simulink model "Test_Decoder_3_to_8"  (R2023a)
settings: Solver=ode45  StartTime=0.0  StopTime=len  RelTol=1e-3  EnableMultiTasking=on
libraries: simulink x2, Decoders_Lib x1
settings Model: Creator=N  LastModifiedBy=Jozko Mrkvicka
settings SolverCC: AlgebraicLoopSolver=TrustRegion
settings DataIOCC: SaveFormat=Array  ReturnWorkspaceOutputs=off
settings OptimizationCC: LifeSpan=inf
settings DebuggingCC: UnconnectedInputMsg=warning  UnconnectedOutputMsg=warning  UnconnectedLineMsg=warning  SFUnexpectedBacktrackingDiag=warning  SFNoUnconditionalDefaultTransitionDiag=warning  SFExecutionAtInitializationDiag=none  ArithmeticOperatorsInVariantConditions=warning
settings HardwareCC: ProdWordSize=32
settings SFSimCC: SimUseLocalCustomCode=off  CustomCodeUndefinedFunction=UseInterfaceOnly
settings RTWCC: RTWUseLocalCustomCode=off
settings CodeAppCC: StateflowObjectComments=on
settings GRTTargetCC: TargetLangStandard=C89/C90 (ANSI)
settings ConfigComp: CovMetricSettings=dw  CovSaveCumulativeToWorkspaceVar=on  CovSaveSingleToWorkspaceVar=on  CovExternalEMLEnable=off

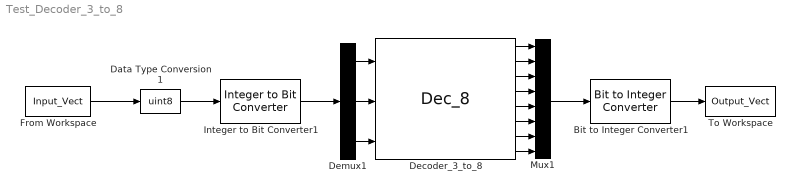
== system Test_Decoder_3_to_8 ==
  Bit to Integer Converter1 : simulink/Logic and Bit Operations/Bit to Integer Converter  nbits=8  bitOrder=MSB first  signedOutputValues=Unsigned  outDtype=uint8  outDtypeSigned=Inherit via internal rule
      settings: LibrarySourceBlock=|
      | commutil2/Bit to Integer
      | Converter
  Data Type Conversion1 : DataTypeConversion  OutDataTypeStr=uint8  SaturateOnIntegerOverflow=off  RndMeth=Floor
  Decoder_3_to_8 : Decoders_Lib/Dec_8  SystemSampleTime=-1  VariantActivationTime=update diagram  Latency=0  AutoFrameSizeCalculation=off
  Demux1 : Demux  Outputs=3
  From Workspace : FromWorkspace  VariableName=Input_Vect  SampleTime=1  Interpolate=off  ZeroCross=off  OutputAfterFinalValue=Holding final value
  Integer to Bit Converter1 : simulink/Logic and Bit Operations/Integer to Bit Converter  nbits=3  signedInputValues=Unsigned  bitOrder=MSB first  outDtype=uint8
      settings: LibrarySourceBlock=|
      | commutil2/Integer to Bit
      | Converter
  Mux1 : Mux  Inputs=8
  To Workspace : ToWorkspace  VariableName=Output_Vect  SampleTime=1
  wires:
  Decoder_3_to_8/1 -> Mux1/1
  Decoder_3_to_8/8 -> Mux1/8
  Decoder_3_to_8/7 -> Mux1/7
  Decoder_3_to_8/6 -> Mux1/6
  Decoder_3_to_8/5 -> Mux1/5
  Decoder_3_to_8/4 -> Mux1/4
  Decoder_3_to_8/3 -> Mux1/3
  Decoder_3_to_8/2 -> Mux1/2
  Mux1/1 -> Bit to Integer Converter1/1
  Demux1/2 -> Decoder_3_to_8/2
  Demux1/3 -> Decoder_3_to_8/3
  Demux1/1 -> Decoder_3_to_8/1
  Integer to Bit Converter1/1 -> Demux1/1
  Data Type Conversion1/1 -> Integer to Bit Converter1/1
  From Workspace/1 -> Data Type Conversion1/1
  Bit to Integer Converter1/1 -> To Workspace/1
